simulink library "Input_Cotton_Oil"  (Simulink 8.2)
settings: Solver=ode45  StartTime=0.0  StopTime=10.0  RelTol=1e-3
settings Model: Creator=lena.frank  LastModifiedBy=drhf

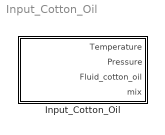
== system Input_Cotton_Oil ==
  Input_Cotton_Oil : Subsystem  mask(Input_Cotton_Oil){T=20, p=1e5}
      mask prompts: T "temperature (scalar or vector) [°C]"; p "pressure [Pa]"
      mask help: Input block for the material "Cotton Oil". The relevant inputs for the calculation of the block can be specified as parameter in the mask
      mask Help: web(fullfile(path_carnot('help'),'input_material.html'),'-helpbrowser')

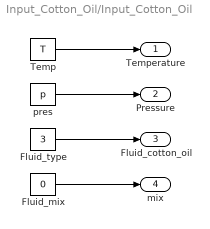
== system Input_Cotton_Oil/Input_Cotton_Oil ==
  Fluid_mix : Constant  Value=0
  Fluid_type : Constant  Value=3
  Temp : Constant  Value=T
  pres : Constant  Value=p
  Temperature : Outport
  Pressure : Outport  Port=2
  Fluid_cotton_oil : Outport  Port=3
  mix : Outport  Port=4
  wires:
  Fluid_mix/1 -> mix/1
  Fluid_type/1 -> Fluid_cotton_oil/1
  Temp/1 -> Temperature/1
  pres/1 -> Pressure/1
